simulink model "quad"  (R2016a)
settings: Solver=FixedStepDiscrete  StartTime=0.0  StopTime=10.0  RelTol=1e-3
libraries: rvs x23
settings Model: Creator=Arthur  LastModifiedBy=arthur
settings DataIOCC: LimitDataPoints=on  SaveFormat=Array
settings DebuggingCC: SolverPrmCheckMsg=warning
settings HardwareCC: ProdBitPerPointer=32  ProdLargestAtomicFloat=None  ProdIntDivRoundTo=Undefined  ProdEndianess=Unspecified  ProdWordSize=32  ProdHWDeviceType=32-bit Generic
settings ModelReferenceCC: PropagateSignalLabelsOutOfModel=off
settings ConfigComp: CovModelRefEnable=Off  CovSFcnEnable=off

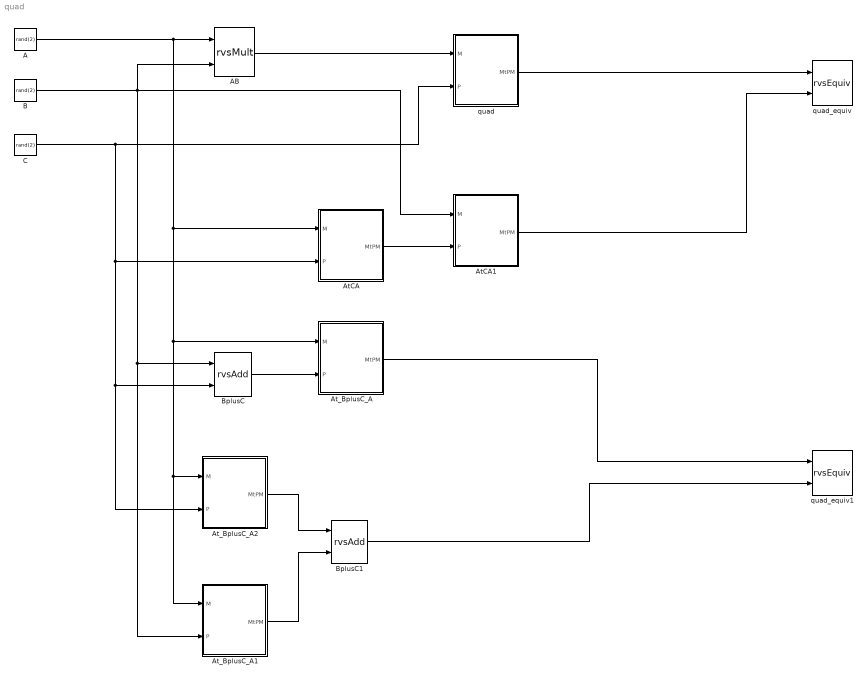
== system quad ==
  A : Constant  Value=rand(2)
  AB : rvs/rvsMult
  AtCA : Subsystem
  AtCA1 : Subsystem
  At_BplusC_A : Subsystem
  At_BplusC_A1 : Subsystem
  At_BplusC_A2 : Subsystem
  B : Constant  Value=rand(2)
  BplusC : rvs/rvsAdd
  BplusC1 : rvs/rvsAdd
  C : Constant  Value=rand(2)
  quad : Subsystem
  quad_equiv : rvs/rvsEquiv  tol=1e-9  nIgnoreSteps=1
  quad_equiv1 : rvs/rvsEquiv  tol=1e-9  nIgnoreSteps=1
  wires:
  C/1 -> At_BplusC_A2/2(P), BplusC/2, AtCA/2(P), quad/2(P)
  A/1 -> At_BplusC_A1/1(M), At_BplusC_A2/1(M), At_BplusC_A/1(M), AtCA/1(M), AB/1
  AB/1 -> quad/1(M)
  quad/1(MtPM) -> quad_equiv/1
  B/1 -> At_BplusC_A1/2(P), BplusC/1, AtCA1/1(M), AB/2
  AtCA1/1(MtPM) -> quad_equiv/2
  AtCA/1(MtPM) -> AtCA1/2(P)
  BplusC/1 -> At_BplusC_A/2(P)
  At_BplusC_A/1(MtPM) -> quad_equiv1/1
  BplusC1/1 -> quad_equiv1/2
  At_BplusC_A2/1(MtPM) -> BplusC1/1
  At_BplusC_A1/1(MtPM) -> BplusC1/2

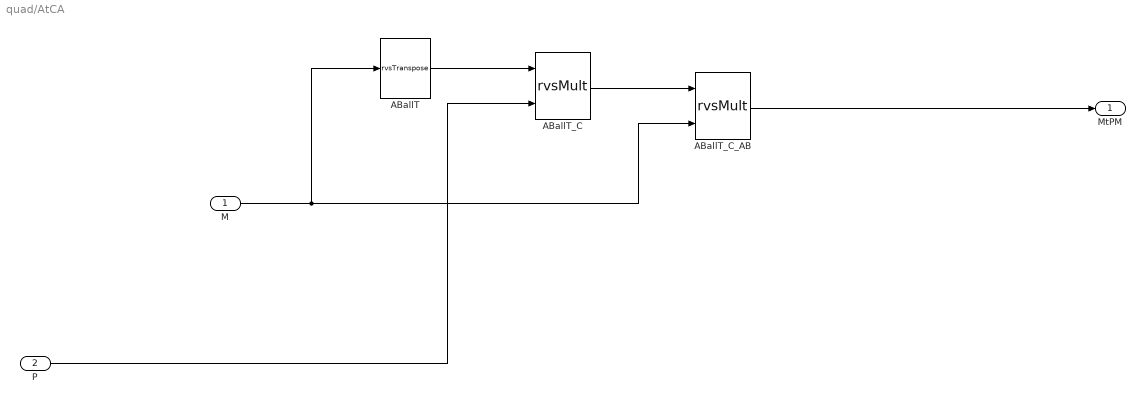
== system quad/AtCA ==
  M : Inport
  P : Inport  Port=2
  ABallT : rvs/rvsTranspose
  ABallT_C : rvs/rvsMult
  ABallT_C_AB : rvs/rvsMult
  MtPM : Outport
  wires:
  ABallT_C_AB/1 -> MtPM/1
  P/1 -> ABallT_C/2
  ABallT/1 -> ABallT_C/1
  M/1 -> ABallT_C_AB/2, ABallT/1
  ABallT_C/1 -> ABallT_C_AB/1

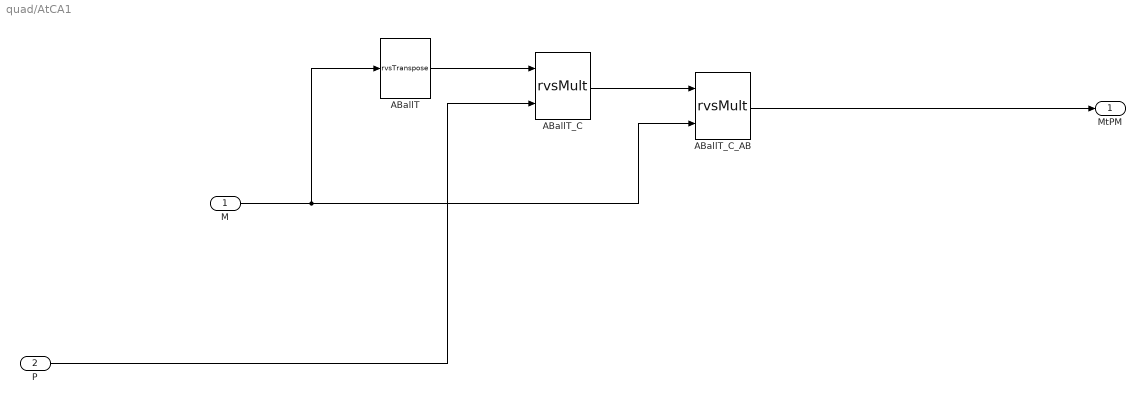
== system quad/AtCA1 ==
  M : Inport
  P : Inport  Port=2
  ABallT : rvs/rvsTranspose
  ABallT_C : rvs/rvsMult
  ABallT_C_AB : rvs/rvsMult
  MtPM : Outport
  wires:
  ABallT_C/1 -> ABallT_C_AB/1
  M/1 -> ABallT/1, ABallT_C_AB/2
  ABallT/1 -> ABallT_C/1
  P/1 -> ABallT_C/2
  ABallT_C_AB/1 -> MtPM/1

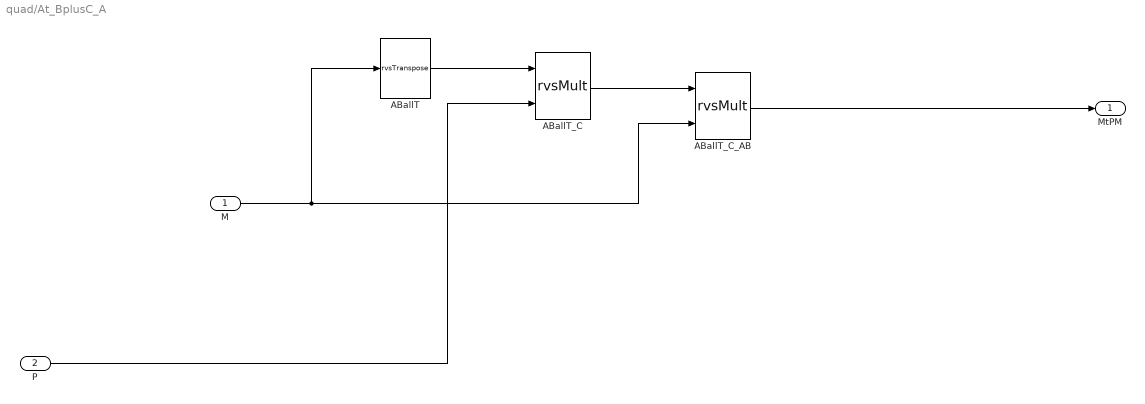
== system quad/At_BplusC_A ==
  M : Inport
  P : Inport  Port=2
  ABallT : rvs/rvsTranspose
  ABallT_C : rvs/rvsMult
  ABallT_C_AB : rvs/rvsMult
  MtPM : Outport
  wires:
  ABallT_C/1 -> ABallT_C_AB/1
  M/1 -> ABallT/1, ABallT_C_AB/2
  ABallT/1 -> ABallT_C/1
  P/1 -> ABallT_C/2
  ABallT_C_AB/1 -> MtPM/1

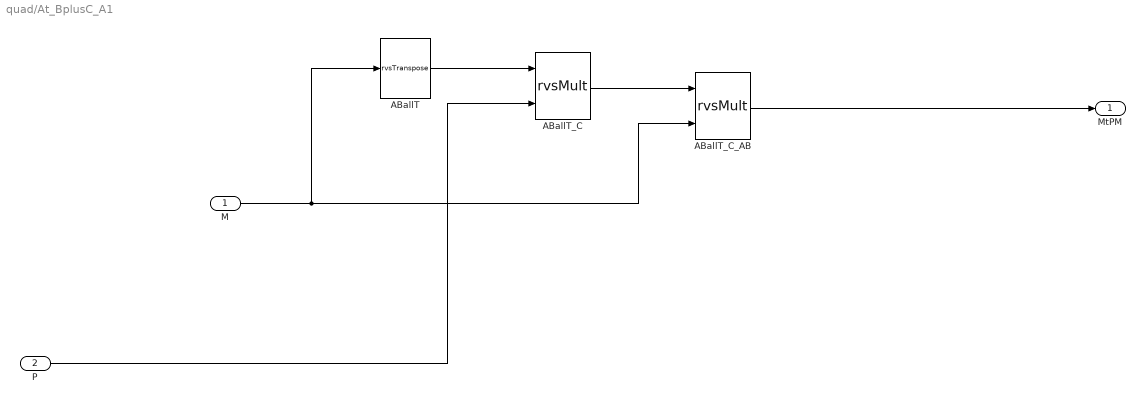
== system quad/At_BplusC_A1 ==
  M : Inport
  P : Inport  Port=2
  ABallT : rvs/rvsTranspose
  ABallT_C : rvs/rvsMult
  ABallT_C_AB : rvs/rvsMult
  MtPM : Outport
  wires:
  ABallT_C_AB/1 -> MtPM/1
  P/1 -> ABallT_C/2
  ABallT/1 -> ABallT_C/1
  M/1 -> ABallT_C_AB/2, ABallT/1
  ABallT_C/1 -> ABallT_C_AB/1

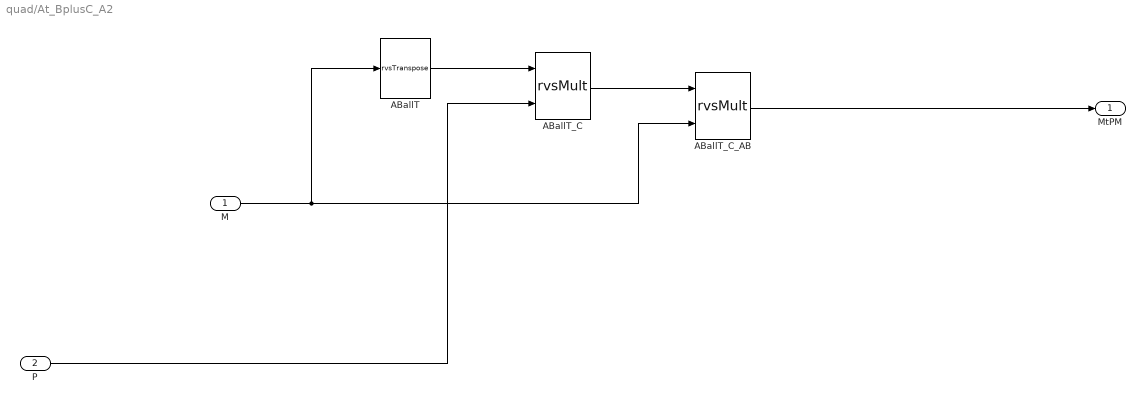
== system quad/At_BplusC_A2 ==
  M : Inport
  P : Inport  Port=2
  ABallT : rvs/rvsTranspose
  ABallT_C : rvs/rvsMult
  ABallT_C_AB : rvs/rvsMult
  MtPM : Outport
  wires:
  ABallT_C/1 -> ABallT_C_AB/1
  M/1 -> ABallT/1, ABallT_C_AB/2
  ABallT/1 -> ABallT_C/1
  P/1 -> ABallT_C/2
  ABallT_C_AB/1 -> MtPM/1

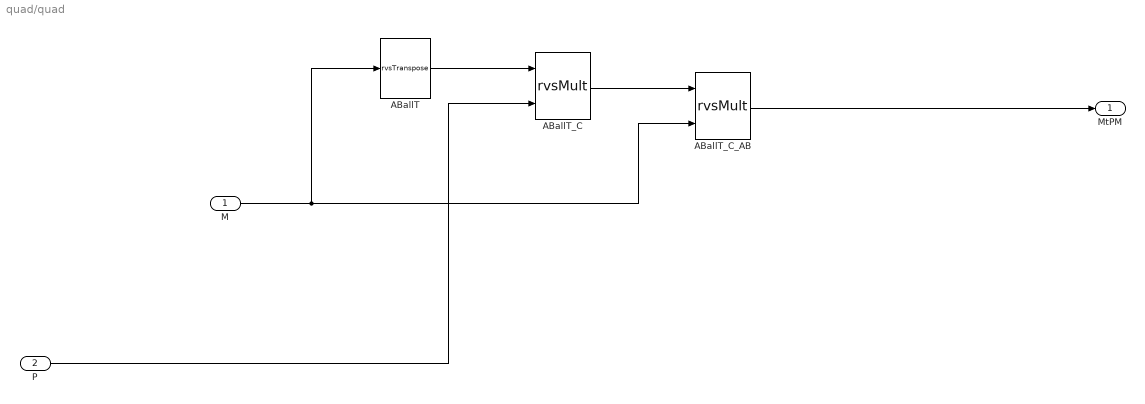
== system quad/quad ==
  M : Inport
  P : Inport  Port=2
  ABallT : rvs/rvsTranspose
  ABallT_C : rvs/rvsMult
  ABallT_C_AB : rvs/rvsMult
  MtPM : Outport
  wires:
  ABallT_C/1 -> ABallT_C_AB/1
  M/1 -> ABallT/1, ABallT_C_AB/2
  ABallT/1 -> ABallT_C/1
  P/1 -> ABallT_C/2
  ABallT_C_AB/1 -> MtPM/1
